simulink model "dpf_regeneration_MIL_SIL_1"  (R2018a)
settings: Solver=FixedStepDiscrete  StartTime=0.0  StopTime=12  FixedStep=1  RelTol=1e-3
settings Model: Creator=admin  LastModifiedBy=admin
settings DataIOCC: ReturnWorkspaceOutputs=on
settings SFSimCC: SimUseLocalCustomCode=on
settings RTWCC: RTWUseLocalCustomCode=on
settings ConfigComp: CovEnable=on  RecordCoverage=on  CovMetricSettings=dcmw  CovHtmlReporting=on  CovModelRefEnable=on  DVMode=DesignErrorDetection  DVTestSuiteOptimization=CombinedObjectives (Nonlinear Extended)  DVDetectDeadLogic=on  DVDetectActiveLogic=on  DVDetectOutOfBounds=on  DVRebuildModelRepresentation=Always

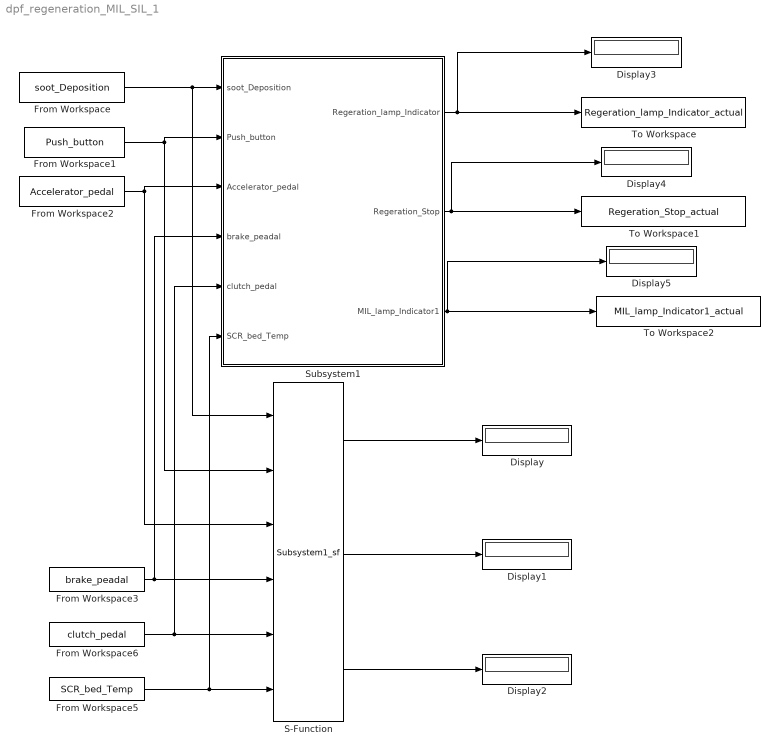
== system dpf_regeneration_MIL_SIL_1 ==
  Display{,1..5} (6 alike) : Display
  From Workspace : FromWorkspace  VariableName=soot_Deposition  SampleTime=0
  From Workspace1 : FromWorkspace  VariableName=Push_button  SampleTime=0
  From Workspace2 : FromWorkspace  VariableName=Accelerator_pedal  SampleTime=0
  From Workspace3 : FromWorkspace  VariableName=brake_peadal  SampleTime=0
  From Workspace5 : FromWorkspace  VariableName=SCR_bed_Temp  SampleTime=0
  From Workspace6 : FromWorkspace  VariableName=clutch_pedal  SampleTime=0
  S-Function : S-Function  FunctionName=Subsystem1_sf  SFunctionDeploymentMode=off  EnableBusSupport=off  SFcnStateName=DWORK0
      settings: SFcnIsStateOwnerBlock=on
  Subsystem1 : Subsystem  TreatAsAtomicUnit=on
  To Workspace : ToWorkspace  VariableName=Regeration_lamp_Indicator_actual  SaveFormat=Timeseries  SampleTime=-1
  To Workspace1 : ToWorkspace  VariableName=Regeration_Stop_actual  SaveFormat=Timeseries  SampleTime=-1
  To Workspace2 : ToWorkspace  VariableName=MIL_lamp_Indicator1_actual  SaveFormat=Timeseries  SampleTime=-1
  wires:
  From Workspace/1 -> S-Function/1, Subsystem1/1(soot_Deposition)
  From Workspace2/1 -> Subsystem1/3(Accelerator_pedal), S-Function/3
  From Workspace1/1 -> Subsystem1/2(Push_button), S-Function/2
  S-Function/3 -> Display2/1
  S-Function/1 -> Display/1
  S-Function/2 -> Display1/1
  From Workspace3/1 -> Subsystem1/4("brake_peadal "), S-Function/4
  From Workspace5/1 -> Subsystem1/6(SCR_bed_Temp), S-Function/6
  From Workspace6/1 -> Subsystem1/5(clutch_pedal), S-Function/5
  Subsystem1/3(MIL_lamp_Indicator1) -> Display5/1, To Workspace2/1
  Subsystem1/2(Regeration_Stop) -> Display4/1, To Workspace1/1
  Subsystem1/1(Regeration_lamp_Indicator) -> Display3/1, To Workspace/1

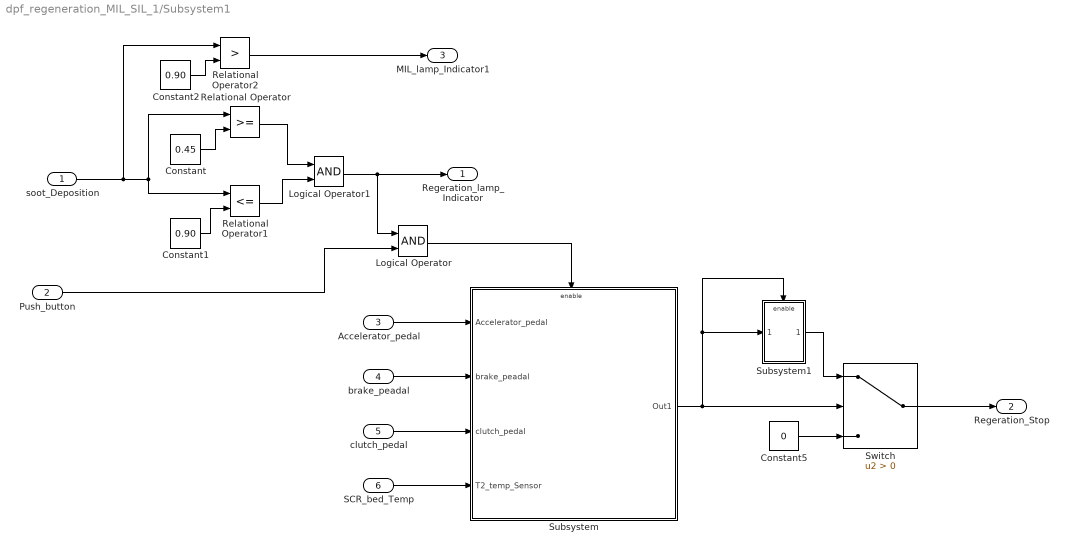
== system dpf_regeneration_MIL_SIL_1/Subsystem1 ==
  soot_Deposition : Inport
  Push_button : Inport  Port=2
  Accelerator_pedal : Inport  Port=3
  "brake_peadal " : Inport  Port=4
  clutch_pedal : Inport  Port=5
  SCR_bed_Temp : Inport  Port=6
  Constant : Constant  Value=0.45
  Constant1 : Constant  Value=0.90
  Constant2 : Constant  Value=0.90
  Constant5 : Constant  Value=0
  Logical Operator : Logic  AllPortsSameDT=off  OutDataTypeStr=boolean
  Logical Operator1 : Logic  AllPortsSameDT=off  OutDataTypeStr=boolean
  Relational Operator : RelationalOperator  OutDataTypeStr=boolean  RndMeth=Simplest
  Relational Operator1 : RelationalOperator  Operator=<=  OutDataTypeStr=boolean  RndMeth=Simplest
  Relational Operator2 : RelationalOperator  Operator=>  OutDataTypeStr=boolean  RndMeth=Simplest
  Subsystem : Subsystem
  Subsystem1 : Subsystem
  Switch : Switch  Criteria=u2 > Threshold
  Regeration_lamp_Indicator : Outport
  Regeration_Stop : Outport  Port=2
  MIL_lamp_Indicator1 : Outport  Port=3
  wires:
  soot_Deposition/1 -> Relational Operator2/1, Relational Operator1/1, Relational Operator/1
  clutch_pedal/1 -> Subsystem/3(clutch_pedal)
  Logical Operator1/1 -> Logical Operator/1, Regeration_lamp_Indicator/1
  Push_button/1 -> Logical Operator/2
  SCR_bed_Temp/1 -> Subsystem/4(T2_temp_Sensor)
  "brake_peadal "/1 -> Subsystem/2("brake_peadal ")
  Constant/1 -> Relational Operator/2
  Constant1/1 -> Relational Operator1/2
  Accelerator_pedal/1 -> Subsystem/1(Accelerator_pedal)
  Logical Operator/1 -> Subsystem/Enable
  Constant5/1 -> Switch/3
  Switch/1 -> Regeration_Stop/1
  Relational Operator/1 -> Logical Operator1/1
  Relational Operator1/1 -> Logical Operator1/2
  Subsystem/1(Out1) -> Switch/2, Subsystem1/Enable, Subsystem1/1(In1)
  Subsystem1/1(Out1) -> Switch/1
  Constant2/1 -> Relational Operator2/2
  Relational Operator2/1 -> MIL_lamp_Indicator1/1

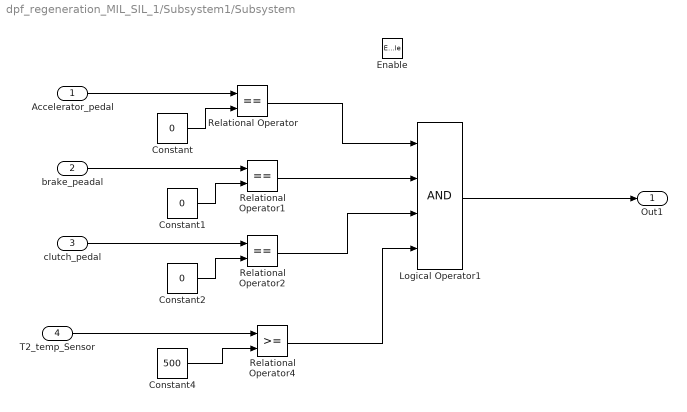
== system dpf_regeneration_MIL_SIL_1/Subsystem1/Subsystem ==
  Accelerator_pedal : Inport
  "brake_peadal " : Inport  Port=2
  clutch_pedal : Inport  Port=3
  T2_temp_Sensor : Inport  Port=4
  Enable : EnablePort  StatesWhenEnabling=reset
  Constant : Constant  Value=0
  Constant1 : Constant  Value=0
  Constant2 : Constant  Value=0
  Constant4 : Constant  Value=500
  Logical Operator1 : Logic  Inputs=4  AllPortsSameDT=off  OutDataTypeStr=boolean
  Relational Operator : RelationalOperator  Operator===  OutDataTypeStr=boolean  RndMeth=Simplest
  Relational Operator1 : RelationalOperator  Operator===  OutDataTypeStr=boolean  RndMeth=Simplest
  Relational Operator2 : RelationalOperator  Operator===  OutDataTypeStr=boolean  RndMeth=Simplest
  Relational Operator4 : RelationalOperator  OutDataTypeStr=boolean  RndMeth=Simplest
  Out1 : Outport
  wires:
  Constant/1 -> Relational Operator/2
  Accelerator_pedal/1 -> Relational Operator/1
  "brake_peadal "/1 -> Relational Operator1/1
  Constant1/1 -> Relational Operator1/2
  Constant2/1 -> Relational Operator2/2
  clutch_pedal/1 -> Relational Operator2/1
  Relational Operator/1 -> Logical Operator1/1
  Relational Operator1/1 -> Logical Operator1/2
  Relational Operator2/1 -> Logical Operator1/3
  T2_temp_Sensor/1 -> Relational Operator4/1
  Constant4/1 -> Relational Operator4/2
  Logical Operator1/1 -> Out1/1
  Relational Operator4/1 -> Logical Operator1/4

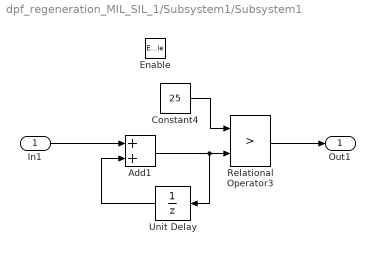
== system dpf_regeneration_MIL_SIL_1/Subsystem1/Subsystem1 ==
  In1 : Inport
  Enable : EnablePort  StatesWhenEnabling=reset
  Add1 : Sum  OutDataTypeStr=int8
  Constant4 : Constant  Value=25
  Relational Operator3 : RelationalOperator  Operator=>  OutDataTypeStr=boolean  RndMeth=Simplest
  Unit Delay : UnitDelay  SampleTime=-1  HasFrameUpgradeWarning=on
  Out1 : Outport
  wires:
  Add1/1 -> Unit Delay/1, Relational Operator3/2
  Relational Operator3/1 -> Out1/1
  Unit Delay/1 -> Add1/2
  Constant4/1 -> Relational Operator3/1
  In1/1 -> Add1/1
